simulink model "part3"  (R2018a)
settings: Solver=VariableStepAuto  StartTime=0.0  StopTime=10  RelTol=1e-3
undefined symbols (not defined in the file): D0, D1, D10, D11, D12, D13, D2, D3, D4, D5, D6, D7, D8, D9, PTA0, PTA1, PTA2, PTB23, PTB9, PTC16, PTC17, PTC2, PTC3, PTC4, PTD0, PTD1, PTD2, PTD3
libraries: frdmk64flib x14
settings Model: Creator=hank_  LastModifiedBy=hank_

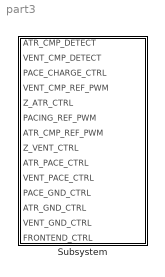
== system part3 ==
  Subsystem : Subsystem

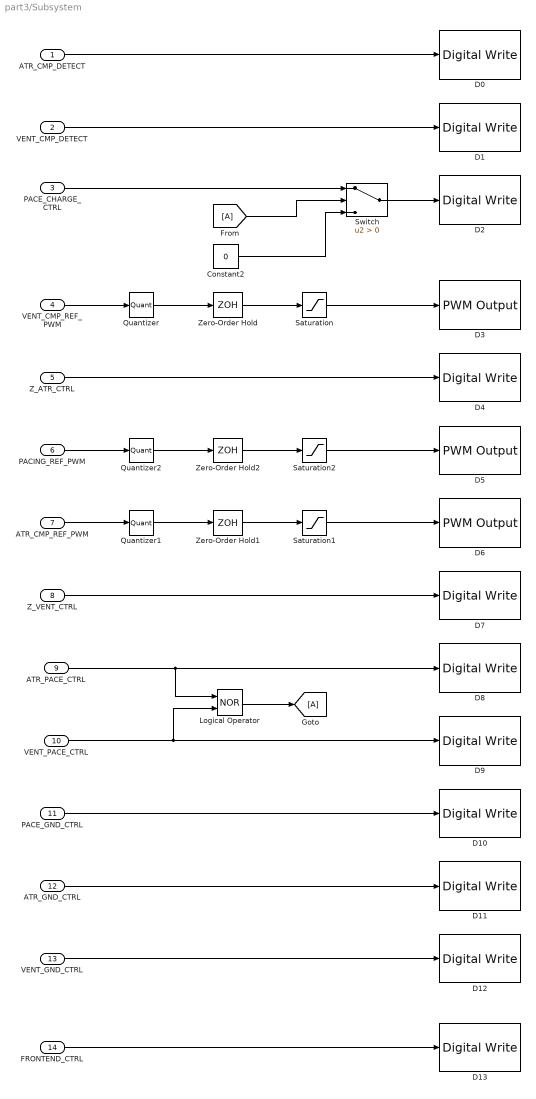
== system part3/Subsystem ==
  ATR_CMP_DETECT : Inport  OutDataTypeStr=boolean
  VENT_CMP_DETECT : Inport  Port=2  OutDataTypeStr=boolean
  PACE_CHARGE_CTRL : Inport  Port=3  OutDataTypeStr=boolean
  VENT_CMP_REF_PWM : Inport  Port=4  OutDataTypeStr=double
  Z_ATR_CTRL : Inport  Port=5  OutDataTypeStr=boolean
  PACING_REF_PWM : Inport  Port=6  OutDataTypeStr=double
  ATR_CMP_REF_PWM : Inport  Port=7  OutDataTypeStr=double
  Z_VENT_CTRL : Inport  Port=8  OutDataTypeStr=boolean
  ATR_PACE_CTRL : Inport  Port=9  OutDataTypeStr=boolean
  VENT_PACE_CTRL : Inport  Port=10  OutDataTypeStr=boolean
  PACE_GND_CTRL : Inport  Port=11  OutDataTypeStr=boolean
  ATR_GND_CTRL : Inport  Port=12  OutDataTypeStr=boolean
  VENT_GND_CTRL : Inport  Port=13  OutDataTypeStr=boolean
  FRONTEND_CTRL : Inport  Port=14  OutDataTypeStr=boolean
  Constant2 : Constant  Value=0  OutDataTypeStr=boolean
  D0 : frdmk64flib/Digital Write  Whichpin=PTC16 (D0)
      settings: SourceProductName=Simulink Coder Support Package for NXP FRDM-K64F Board
  D1 : frdmk64flib/Digital Write  Whichpin=PTC17 (D1)
      settings: SourceProductName=Simulink Coder Support Package for NXP FRDM-K64F Board
  D10 : frdmk64flib/Digital Write  Whichpin=PTD0 (D10)
      settings: SourceProductName=Simulink Coder Support Package for NXP FRDM-K64F Board
  D11 : frdmk64flib/Digital Write  Whichpin=PTD2 (D11)
      settings: SourceProductName=Simulink Coder Support Package for NXP FRDM-K64F Board
  D12 : frdmk64flib/Digital Write  Whichpin=PTD3 (D12)
      settings: SourceProductName=Simulink Coder Support Package for NXP FRDM-K64F Board
  D13 : frdmk64flib/Digital Write  Whichpin=PTD1 (D13)
      settings: SourceProductName=Simulink Coder Support Package for NXP FRDM-K64F Board
  D2 : frdmk64flib/Digital Write  Whichpin=PTB9 (D2)
      settings: SourceProductName=Simulink Coder Support Package for NXP FRDM-K64F Board
  D3 : frdmk64flib/PWM Output  Whichpin=PTA1 (D3)  InitialFrequency=916  InitialDutyCycle=0
      settings: SourceProductName=Simulink Coder Support Package for NXP FRDM-K64F Board
  D4 : frdmk64flib/Digital Write  Whichpin=PTB23 (D4)
      settings: SourceProductName=Simulink Coder Support Package for NXP FRDM-K64F Board
  D5 : frdmk64flib/PWM Output  Whichpin=PTA2 (D5)  InitialFrequency=916  InitialDutyCycle=0
      settings: SourceProductName=Simulink Coder Support Package for NXP FRDM-K64F Board
  D6 : frdmk64flib/PWM Output  Whichpin=PTC2 (D6)  InitialFrequency=916  InitialDutyCycle=0
      settings: SourceProductName=Simulink Coder Support Package for NXP FRDM-K64F Board
  D7 : frdmk64flib/Digital Write  Whichpin=PTC3 (D7)
      settings: SourceProductName=Simulink Coder Support Package for NXP FRDM-K64F Board
  "D8 " : frdmk64flib/Digital Write  Whichpin=PTA0 (D8)
      settings: SourceProductName=Simulink Coder Support Package for NXP FRDM-K64F Board
  D9 : frdmk64flib/Digital Write  Whichpin=PTC4 (D9)
      settings: SourceProductName=Simulink Coder Support Package for NXP FRDM-K64F Board
  Logical Operator : Logic  Operator=NOR  AllPortsSameDT=off  OutDataTypeStr=boolean
  Quantizer : Quantizer  QuantizationInterval=0.01
  Quantizer1 : Quantizer  QuantizationInterval=0.01
  Quantizer2 : Quantizer  QuantizationInterval=0.01
  Saturation : Saturate  UpperLimit=100  LowerLimit=0
  Saturation1 : Saturate  UpperLimit=100  LowerLimit=0
  Saturation2 : Saturate  UpperLimit=100  LowerLimit=0
  Switch : Switch  Criteria=u2 > Threshold
  Zero-Order Hold : ZeroOrderHold  SampleTime=0.01
  Zero-Order Hold1 : ZeroOrderHold  SampleTime=0.01
  Zero-Order Hold2 : ZeroOrderHold  SampleTime=0.01
  wires:
  ATR_CMP_DETECT/1 -> D0/1
  VENT_CMP_DETECT/1 -> D1/1
  Z_ATR_CTRL/1 -> D4/1
  Z_VENT_CTRL/1 -> D7/1
  VENT_PACE_CTRL/1 -> D9/1, Logical Operator/2
  PACE_GND_CTRL/1 -> D10/1
  ATR_GND_CTRL/1 -> D11/1
  VENT_GND_CTRL/1 -> D12/1
  FRONTEND_CTRL/1 -> D13/1
  ATR_PACE_CTRL/1 -> "D8 "/1, Logical Operator/1
  Switch/1 -> D2/1
  PACE_CHARGE_CTRL/1 -> Switch/1
  Constant2/1 -> Switch/3
  VENT_CMP_REF_PWM/1 -> Quantizer/1
  Quantizer/1 -> Zero-Order Hold/1
  Quantizer1/1 -> Zero-Order Hold1/1
  Zero-Order Hold1/1 -> Saturation1/1
  Saturation1/1 -> D6/1
  ATR_CMP_REF_PWM/1 -> Quantizer1/1
  Zero-Order Hold2/1 -> Saturation2/1
  Saturation2/1 -> D5/1
  Quantizer2/1 -> Zero-Order Hold2/1
  PACING_REF_PWM/1 -> Quantizer2/1
  [A] -> Switch/2
  Logical Operator/1 -> [A]
  Saturation/1 -> D3/1
  Zero-Order Hold/1 -> Saturation/1
